simulink library "mExternalMlib"  (Simulink 8.5)
settings: Solver=ode45  SolverMode=SingleTasking  StartTime=0.0  StopTime=10.0  RelTol=1e-3
settings Model: Creator=shirwani  LastModifiedBy=sbergstr

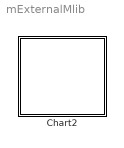
== system mExternalMlib ==
  Chart2 : Stateflow chart  TreatAsAtomicUnit=on

== matlab function Chart2 ==
  data: em2_out function_output double; em2_in function_input double
function em2_out = lib_em2(em2_in)
a = externalmfile(em2_in);
em2_out = em2_in * 2 + a;
